simulink model "local_dp_tug"  (Simulink 10.1)
settings: Solver=ode4  StartTime=0.0  StopTime=1000  FixedStep=1  RelTol=1e-3  EnableMultiTasking=on
PreLoadFcn:
  | load('Initialization_data.mat');
values from neighbouring files (symbols this model uses):
  D1 = [MM(1,1)/100, 0, 0; 0, MM(2,2)/40, 0; 0, 0, MM(3,3)/20]    [initail_data.m]    (also in msfun_backstepping_controller.m = [MM1(1,1)/100, 0, 0; 0, MM1(2,2)/40, 0; 0, 0, MM1(3,3)/20]; temp_code.m = [MM1(1,1)/100, 0, 0; 0, MM1(2,2)/40, 0; 0, 0, MM1(3,3)/20])
  M1 = diag([6.25e5, 6.25e5, 6.25e5*7.5^2])    [initail_data.m]    (also in msfun_backstepping_controller.m; temp_code.m)
  Ma1 = [7.58e4, 0, 0; 0, 3.69e5 -1.4e5; 0, -1.4e5, 8.77e6]    [initail_data.m]    (also in msfun_backstepping_controller.m; temp_code.m)
undefined symbols (not defined in the file or in its folder): magnitude
libraries: simulink x3, simulink_extras x1
settings Model: Creator=Lither  LastModifiedBy=jiang
settings DataIOCC: LimitDataPoints=on
settings OptimizationCC: ExpressionDepthLimit=2147483647
settings DebuggingCC: FcnCallInpInsideContextMsg=warning  StateNameClashWarn=warning
settings ConfigComp: CovSFcnEnable=off

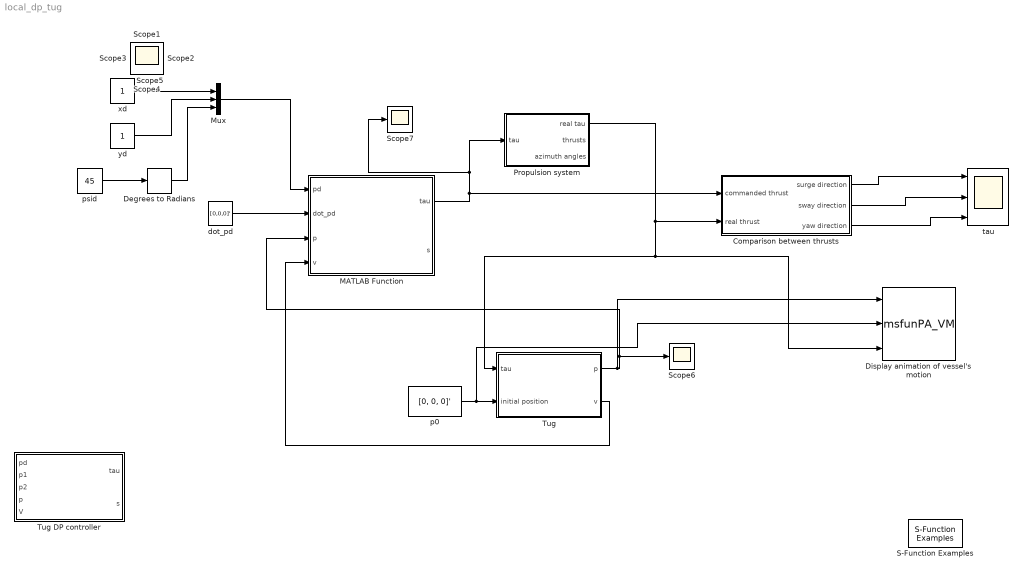
== system local_dp_tug ==
  Comparison between thrusts : Subsystem
  Degrees to Radians : simulink_extras/Transformations/Degrees to Radians
  Display animation of vessel's motion : M-S-Function  FunctionName=msfunPA_VM
  MATLAB Function : MATLAB Function  InitFcn=ei = zeros(3, 1);  TreatAsAtomicUnit=on  mask{Kd=diag([2.5, 2.5, 2])*1, Ki=diag([0.1, 0.1, 0.05])*1, Gama=diag([0.7, 0.7, 0.7])*1}
  Mux : Mux  Inputs=3
  Propulsion system : Subsystem  mask{f0=[100;100;100], a0=[-50;60;-100], u0=[1; 1; 1], wa=on}
      mask prompts: f0 "Initial values of thrusts"; a0 "Initial values of azimuth angles"; u0 "Thruster utilization"; wa "Show animation of thrust and azimuth angle"
  S-Function Examples : simulink/User-Defined Functions/S-Function Examples
      settings: SourceProductBaseCode=SL
  Scope{,1..7} (8 alike) : Scope
  Tug : Subsystem  mask{wv=on}
      mask prompts: wv "Display animation of the vessel's motion"
  Tug DP controller : Subsystem  mask(Nonlinear DP Controller){K=diag([1, 1, 1])/10, Ki=diag([1, 1, 1]), Gama=diag([1, 1, 1])}
      mask prompts: K "Proportional Gain Matrix: K"; Ki "Integral Gain Matrix: Ki"
      mask help: PID controller for Set-Point Reulation in Surge, Sway and Yaw
      mask Help:
      | The nonlinear  PID controller uses the rotation matrix in yaw for proper scaling of the surge, sway and yaw gains as a function of the yaw angle.
      | INPUTS: (1) eta_ref, (2) eta, (3) nu. OUPUTS: (1) tau.
      mask Display: disp('BS controller')
  dot_pd : Constant  Value=[0,0,0]'
  p0 : Constant  Value=[0, 0, 0]'
  psid : Constant  Value=45
  tau : Scope  NumInputPorts=3
  xd : Constant
  yd : Constant
  wires:
  xd/1 -> Mux/1
  yd/1 -> Mux/2
  Mux/1 -> MATLAB Function/1(pd)
  Tug/1(p) -> Display animation of vessel's motion/1, MATLAB Function/3(p), Scope6/1
  psid/1 -> Degrees to Radians/1
  Degrees to Radians/1 -> Mux/3
  p0/1 -> Display animation of vessel's motion/2, Tug/2(initial position)
  MATLAB Function/1(tau) -> Scope7/1, Propulsion system/1(tau), Comparison between thrusts/1(commanded thrust)
  Tug/2(v) -> MATLAB Function/4(v)
  Comparison between thrusts/2(sway direction) -> tau/2
  Comparison between thrusts/1(surge direction) -> tau/1
  Comparison between thrusts/3(yaw direction) -> tau/3
  Propulsion system/1(real tau) -> Display animation of vessel's motion/3, Tug/1(tau), Comparison between thrusts/2(real thrust)
  dot_pd/1 -> MATLAB Function/2(dot_pd)

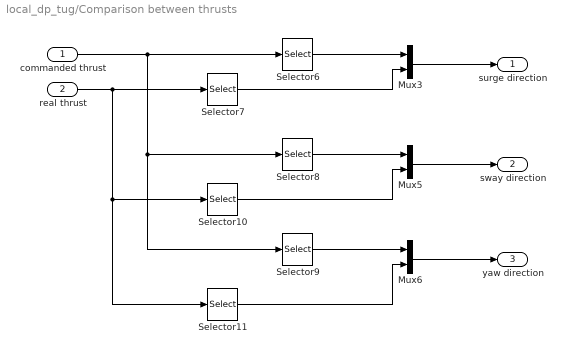
== system local_dp_tug/Comparison between thrusts ==
  commanded thrust : Inport
  real thrust : Inport  Port=2
  Mux3 : Mux  Inputs=2
  Mux5 : Mux  Inputs=2
  Mux6 : Mux  Inputs=2
  Selector10 : Selector  InputPortWidth=3  IndexOptions=Index vector (dialog)  Indices=[2]  OutputSizes=1
  Selector11 : Selector  InputPortWidth=3  IndexOptions=Index vector (dialog)  Indices=[3]  OutputSizes=1
  Selector6 : Selector  InputPortWidth=3  IndexOptions=Index vector (dialog)  Indices=[1]  OutputSizes=1
  Selector7 : Selector  InputPortWidth=3  IndexOptions=Index vector (dialog)  Indices=[1]  OutputSizes=1
  Selector8 : Selector  InputPortWidth=3  IndexOptions=Index vector (dialog)  Indices=[2]  OutputSizes=1
  Selector9 : Selector  InputPortWidth=3  IndexOptions=Index vector (dialog)  Indices=[3]  OutputSizes=1
  surge direction : Outport
  sway direction : Outport  Port=2
  yaw direction : Outport  Port=3
  wires:
  Selector9/1 -> Mux6/1
  Selector11/1 -> Mux6/2
  Selector10/1 -> Mux5/2
  Selector8/1 -> Mux5/1
  Selector7/1 -> Mux3/2
  Selector6/1 -> Mux3/1
  Mux3/1 -> surge direction/1
  Mux5/1 -> sway direction/1
  Mux6/1 -> yaw direction/1
  commanded thrust/1 -> Selector6/1, Selector8/1, Selector9/1
  real thrust/1 -> Selector7/1, Selector10/1, Selector11/1

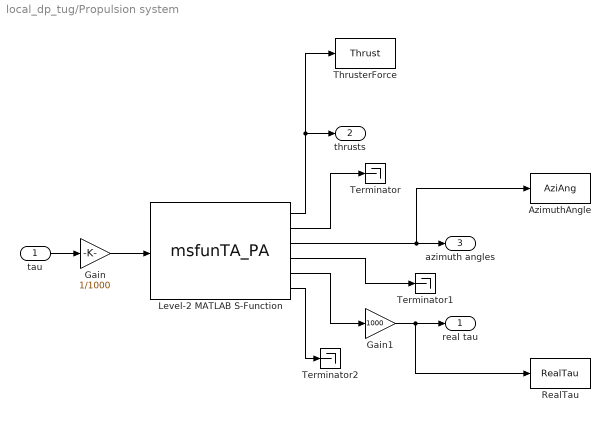
== system local_dp_tug/Propulsion system ==
  tau : Inport
  AzimuthAngle : ToWorkspace  VariableName=AziAng  SampleTime=-1
  Gain : Gain  Gain=1/1000
  Gain1 : Gain  Gain=1000
  Level-2 MATLAB S-Function : M-S-Function  FunctionName=msfunTA_PA  Parameters=f0,a0,wa
  RealTau : ToWorkspace  VariableName=RealTau  SampleTime=-1
  Terminator : Terminator
  Terminator1 : Terminator
  Terminator2 : Terminator
  ThrusterForce : ToWorkspace  VariableName=Thrust  SampleTime=-1
  real tau : Outport
  thrusts : Outport  Port=2
  azimuth angles : Outport  Port=3
  wires:
  tau/1 -> Gain/1
  Level-2 MATLAB S-Function/2 -> Terminator/1
  Level-2 MATLAB S-Function/3 -> AzimuthAngle/1, azimuth angles/1
  Level-2 MATLAB S-Function/4 -> Terminator1/1
  Level-2 MATLAB S-Function/5 -> Gain1/1
  Level-2 MATLAB S-Function/6 -> Terminator2/1
  Level-2 MATLAB S-Function/1 -> ThrusterForce/1, thrusts/1
  Gain/1 -> Level-2 MATLAB S-Function/1
  Gain1/1 -> RealTau/1, real tau/1

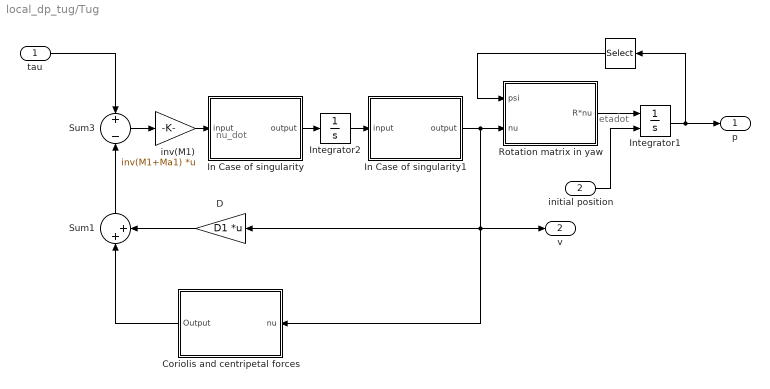
== system local_dp_tug/Tug ==
  note: nu_dot
  note: etadot
  tau : Inport
  initial position : Inport  Port=2
  " " : Selector  InputPortWidth=3  IndexOptions=Index vector (dialog)  Indices=[3]  OutputSizes=1
  Coriolis and centripetal forces : Subsystem
  D : Gain  Gain=D1  Multiplication=Matrix(K*u)  SaturateOnIntegerOverflow=on  OutDataTypeStr=Inherit: Same as input  ParamDataTypeStr=Inherit: Same as input
  In Case of singularity : Subsystem
  In Case of singularity1 : Subsystem
  Integrator1 : Integrator  InitialConditionSource=external  InitialCondition=1.05
  Integrator2 : Integrator
  Rotation matrix in yaw : Subsystem
  Sum1 : Sum  Inputs=|++  InputSameDT=on  SaturateOnIntegerOverflow=on  OutDataTypeStr=Inherit: Same as first input
  Sum3 : Sum  Inputs=+-  InputSameDT=on  SaturateOnIntegerOverflow=on  OutDataTypeStr=Inherit: Same as first input
  inv(M1) : Gain  Gain=inv(M1+Ma1)  Multiplication=Matrix(K*u)  SaturateOnIntegerOverflow=on  OutDataTypeStr=Inherit: Same as input  ParamDataTypeStr=Inherit: Same as input
  p : Outport
  v : Outport  Port=2
  wires:
  Sum3/1 -> inv(M1)/1
  inv(M1)/1 -> In Case of singularity/1(input)
  Rotation matrix in yaw/1(R*nu) -> Integrator1/1
  Integrator1/1 -> p/1, " "/1
  " "/1 -> Rotation matrix in yaw/1(psi)
  tau/1 -> Sum3/1
  initial position/1 -> Integrator1/2
  Integrator2/1 -> In Case of singularity1/1(input)
  In Case of singularity/1(output) -> Integrator2/1
  In Case of singularity1/1(output) -> Rotation matrix in yaw/2(nu), D/1, Coriolis and centripetal forces/1(nu), v/1
  D/1 -> Sum1/2
  Coriolis and centripetal forces/1(Output) -> Sum1/1
  Sum1/1 -> Sum3/2

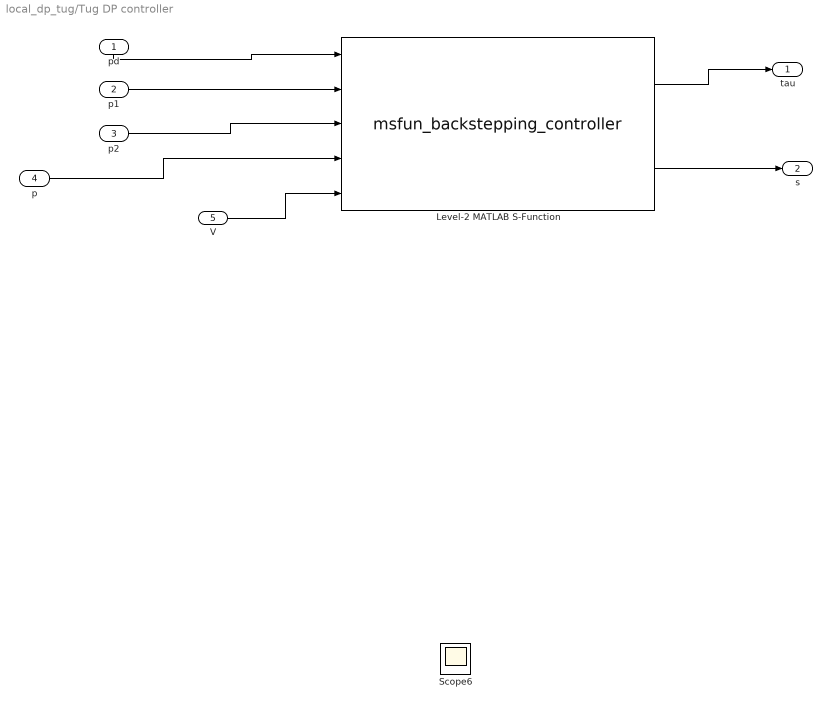
== system local_dp_tug/Tug DP controller ==
  pd : Inport
  p1 : Inport  Port=2
  p2 : Inport  Port=3
  p : Inport  Port=4
  V : Inport  Port=5
  Level-2 MATLAB S-Function : M-S-Function  FunctionName=msfun_backstepping_controller  Parameters=K, Ki, Gama
      settings: AttributesFormatString=|
      | %<Mask>
      | %<Parameters>
      | %<Mask>
  Scope6 : Scope
  tau : Outport
  s : Outport  Port=2
  wires:
  p/1 -> Level-2 MATLAB S-Function/4
  V/1 -> Level-2 MATLAB S-Function/5
  pd/1 -> Level-2 MATLAB S-Function/1
  p1/1 -> Level-2 MATLAB S-Function/2
  p2/1 -> Level-2 MATLAB S-Function/3
  Level-2 MATLAB S-Function/1 -> tau/1
  Level-2 MATLAB S-Function/2 -> s/1

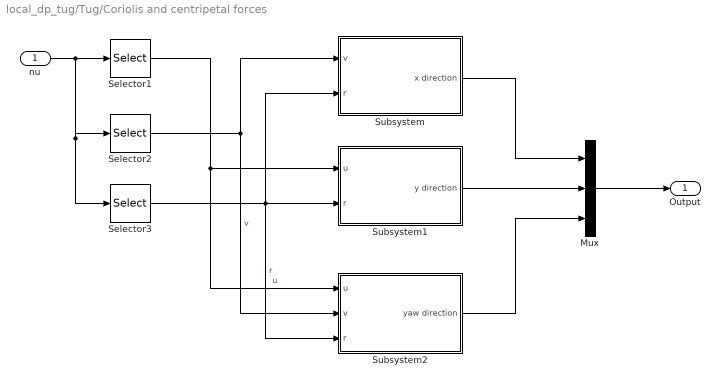
== system local_dp_tug/Tug/Coriolis and centripetal forces ==
  nu : Inport
  Mux : Mux  Inputs=3
  Selector1 : Selector  InputPortWidth=3  IndexOptions=Index vector (dialog)  Indices=[1 ]  OutputSizes=1
  Selector2 : Selector  InputPortWidth=3  IndexOptions=Index vector (dialog)  Indices=[2]  OutputSizes=1
  Selector3 : Selector  InputPortWidth=3  IndexOptions=Index vector (dialog)  Indices=[3]  OutputSizes=1
  Subsystem : Subsystem
  Subsystem1 : Subsystem
  Subsystem2 : Subsystem
  Output : Outport
  wires:
  nu/1 -> Selector1/1, Selector2/1, Selector3/1
  Selector2/1 -> Subsystem/1(v), Subsystem2/2(v)  "v"
  Selector3/1 -> Subsystem/2(r), Subsystem1/2(r), Subsystem2/3(r)  "r"
  Selector1/1 -> Subsystem1/1(u), Subsystem2/1(u)  "u"
  Subsystem/1(x direction) -> Mux/1
  Subsystem1/1(y direction) -> Mux/2
  Subsystem2/1(yaw direction) -> Mux/3
  Mux/1 -> Output/1

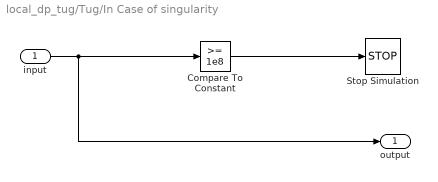
== system local_dp_tug/Tug/In Case of singularity ==
  input : Inport
  Compare To Constant : simulink/Logic and Bit Operations/Compare To Constant  relop=>=  const=1e8  OutDataTypeStr=boolean
  Stop Simulation : Stop
  output : Outport
  wires:
  input/1 -> output/1, Compare To Constant/1
  Compare To Constant/1 -> Stop Simulation/1

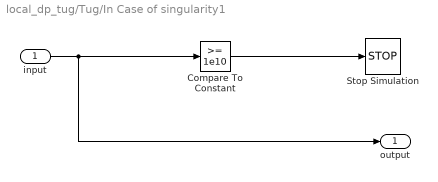
== system local_dp_tug/Tug/In Case of singularity1 ==
  input : Inport
  Compare To Constant : simulink/Logic and Bit Operations/Compare To Constant  relop=>=  const=1e10  OutDataTypeStr=boolean
  Stop Simulation : Stop
  output : Outport
  wires:
  input/1 -> output/1, Compare To Constant/1
  Compare To Constant/1 -> Stop Simulation/1

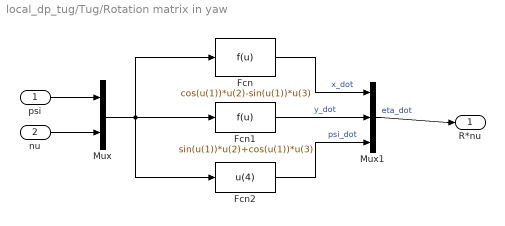
== system local_dp_tug/Tug/Rotation matrix in yaw ==
  psi : Inport
  nu : Inport  Port=2
  Fcn : Fcn  Expr=cos(u(1))*u(2)-sin(u(1))*u(3)
  Fcn1 : Fcn  Expr=sin(u(1))*u(2)+cos(u(1))*u(3)
  Fcn2 : Fcn  Expr=u(4)
  Mux : Mux  Inputs=2
  Mux1 : Mux  Inputs=3
  R*nu : Outport
  wires:
  Mux1/1 -> R*nu/1  "eta_dot"
  Mux/1 -> Fcn/1, Fcn1/1, Fcn2/1
  psi/1 -> Mux/1
  nu/1 -> Mux/2
  Fcn1/1 -> Mux1/2  "y_dot"
  Fcn/1 -> Mux1/1  "x_dot"
  Fcn2/1 -> Mux1/3  "psi_dot"

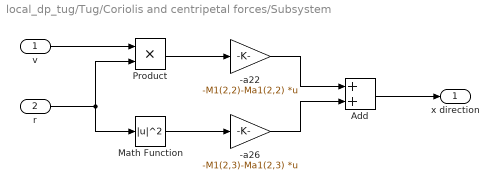
== system local_dp_tug/Tug/Coriolis and centripetal forces/Subsystem ==
  v : Inport
  r : Inport  Port=2
  -a22 : Gain  Gain=-M1(2,2)-Ma1(2,2)  Multiplication=Matrix(K*u)  SaturateOnIntegerOverflow=on  OutDataTypeStr=Inherit: Same as input  ParamDataTypeStr=Inherit: Same as input
  -a26 : Gain  Gain=-M1(2,3)-Ma1(2,3)  Multiplication=Matrix(K*u)  SaturateOnIntegerOverflow=on  OutDataTypeStr=Inherit: Same as input  ParamDataTypeStr=Inherit: Same as input
  Add : Sum
  Math Function : Math  Operator=magnitude^2  SignedPower=on  SaturateOnIntegerOverflow=on
  Product : Product  RndMeth=Zero
  x direction : Outport
  wires:
  v/1 -> Product/1
  r/1 -> Product/2, Math Function/1
  Product/1 -> -a22/1
  Math Function/1 -> -a26/1
  -a22/1 -> Add/1
  -a26/1 -> Add/2
  Add/1 -> x direction/1

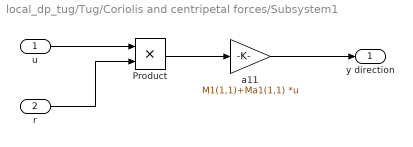
== system local_dp_tug/Tug/Coriolis and centripetal forces/Subsystem1 ==
  u : Inport
  r : Inport  Port=2
  Product : Product  RndMeth=Zero
  a11 : Gain  Gain=M1(1,1)+Ma1(1,1)  Multiplication=Matrix(K*u)  SaturateOnIntegerOverflow=on  OutDataTypeStr=Inherit: Same as input  ParamDataTypeStr=Inherit: Same as input
  y direction : Outport
  wires:
  Product/1 -> a11/1
  r/1 -> Product/2
  u/1 -> Product/1
  a11/1 -> y direction/1

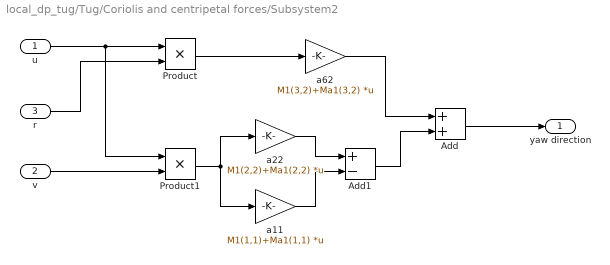
== system local_dp_tug/Tug/Coriolis and centripetal forces/Subsystem2 ==
  u : Inport
  v : Inport  Port=2
  r : Inport  Port=3
  Add : Sum
  Add1 : Sum  Inputs=+-
  Product : Product  RndMeth=Zero
  Product1 : Product  RndMeth=Zero
  a11 : Gain  Gain=M1(1,1)+Ma1(1,1)  Multiplication=Matrix(K*u)  SaturateOnIntegerOverflow=on  OutDataTypeStr=Inherit: Same as input  ParamDataTypeStr=Inherit: Same as input
  a22 : Gain  Gain=M1(2,2)+Ma1(2,2)  Multiplication=Matrix(K*u)  SaturateOnIntegerOverflow=on  OutDataTypeStr=Inherit: Same as input  ParamDataTypeStr=Inherit: Same as input
  a62 : Gain  Gain=M1(3,2)+Ma1(3,2)  Multiplication=Matrix(K*u)  SaturateOnIntegerOverflow=on  OutDataTypeStr=Inherit: Same as input  ParamDataTypeStr=Inherit: Same as input
  yaw direction : Outport
  wires:
  u/1 -> Product/1, Product1/1
  r/1 -> Product/2
  Product/1 -> a62/1
  v/1 -> Product1/2
  Product1/1 -> a22/1, a11/1
  a22/1 -> Add1/1
  a11/1 -> Add1/2
  Add1/1 -> Add/2
  a62/1 -> Add/1
  Add/1 -> yaw direction/1

== matlab function MATLAB Function ==
  settings: updateMethod=DISCRETE
  data: pd input double; tau output double; dot_pd input double; p input double; v input double; s output double
function [tau, s] = bs_constroller(pd, dot_pd, p, v)
% input:
% pd, dot_pd, ddot_pd: 轨迹
% p, v : 实时位置和速度

%output:
% tau: 控制力
% s： 中间变量（速度相关）

persistent ei;
if isempty(ei)  %初始化
    ei = zeros(3, 1);
end

M1 = diag([6.25e5, 6.25e5, 6.25e5*7.5^2]);
Ma1 = [7.58e4, 0, 0; 0, 3.69e5 -1.4e5; 0, -1.4e5, 8.77e6];
MM1 = M1 + Ma1;
D1 = [MM1(1,1)/100, 0, 0; 0, MM1(2,2)/40, 0; 0, 0, MM1(3,3)/20];
%     global ei MM1 D1 
%     ei = 0;

Kd = diag([2.5, 2.5, 2])*1;
Ki = diag([0.1, 0.1, 0.05])*1;
%     Kd = diag([1, 1, 1])*20;
%     Ki = diag([1, 1, 1])*2;
    Gama = diag([1, 1, 1])*0.7;

    ddot_pd = zeros(3, 1);
    
    
    R = rotate_matrix(p);
    dot_R = dot_rotate_matrix(p, v);
    
    p_error = p - pd;
    dot_pr = dot_pd - Gama * p_error;
    ddot_pr = ddot_pd - Gama * (R * v - dot_pd);
    s = R * v -dot_pr;

    ei = ei + p_error * 1; %误差累计，用于积分用
    
    imax = 100;
    for i = 1 : 3
        if ei(i) > imax
            ei(i) = imax;
        end
        if ei(i) < -imax
            ei(i) = -imax;
        end
    end
        
    
    C1 = C_matrix(MM1, v);
    Mp1 = R * MM1 * R';
    Dp1 = R * D1 * R';
    Cp1 = R * (C1 - MM1 * R' * dot_R) * R';
    
    tau = R' * (Mp1 * ddot_pr + Cp1 * dot_pr + Dp1 * dot_pr - Kd * s - Ki * ei);
    
    tau = tau/1e3;
    

end






function R = rotate_matrix(p)
    fai = p(3);
    R = [cos(fai),  -sin(fai),  0;
         sin(fai),  cos(fai),   0;
         0,          0,         1];   
end

function dotR = dot_rotate_matrix(p, v)
    fai = p(3);
    r = v(3);
    dotR = [-sin(fai)*r, -cos(fai)*r, 0;
           cos(fai)*r, -sin(fai)*r, 0;
           0, 0, 0];
end
    
function C = C_matrix(M, v)
    C = [0, 0, -M(2, 2) * v(2) - M(2, 3) * v(3);
        0, 0, M(1, 1) * v(1);
        M(2, 2) * v(2) + M(3, 2) * v(3), -M(1, 1) * v(1), 0];
end
